simulink model "pid_C2000"  (R2018a)
settings: Solver=FixedStepDiscrete  StartTime=0.0  StopTime=Inf  RelTol=1e-3
undefined symbols (not defined in the file): Asymmetric, Up
libraries: c281xlib x2
settings Model: ExtModeTrigDuration=8  Creator=Administrator  LastModifiedBy=Administrator
settings SolverCC: AlgebraicLoopSolver=LineSearch
settings OptimizationCC: DefaultParameterBehavior=Inlined  UseDivisionForNetSlopeComputation=on  UseFloatMulNetSlope=on  DefaultUnderspecifiedDataType=single  InlineInvariantSignals=on  PassReuseOutputArgsAs=Individual arguments  ZeroExternalMemoryAtStartup=off  NoFixptDivByZeroProtection=on  EfficientFloat2IntCast=on  LifeSpan=1  MaxStackSize=512  OptimizeBlockOrder=speed  DifferentSizesBufferReuse=on
settings DebuggingCC: AlgebraicLoopMsg=none  ParameterTunabilityLossMsg=error
settings HardwareCC: ProdBitPerChar=16  ProdBitPerInt=16  ProdBitPerPointer=32  ProdBitPerSizeT=32  ProdBitPerPtrDiffT=32  ProdLargestAtomicInteger=Integer  ProdLargestAtomicFloat=None  ProdWordSize=16  ProdLongLongMode=on  ProdHWDeviceType=Texas Instruments->C2000
settings SFSimCC: MATLABDynamicMemAlloc=off
settings RTWCC: SystemTargetFile=ert.tlc  HardwareBoard=TI F281x  TLCOptions=-aInlineSetEventsForThisBaseRateFcn=TLC_FALSE -aSuppressMultiTaskScheduler=TLC_FALSE -aRateBasedStepFcn=1  TemplateMakefile=ert_default_tmf  GenerateReport=on  Toolchain=Texas Instruments Code Composer Studio (C2000)  IncludeHyperlinkInReport=on  LaunchReport=on  GenerateTraceInfo=on  GenerateTraceReport=on  GenerateTraceReportSl=on  GenerateTraceReportSf=on  GenerateTraceReportEml=on  GenerateCodeMetricsReport=on
settings CodeAppCC: ForceParamTrailComments=on  IgnoreCustomStorageClasses=off  OperatorAnnotations=on  SimulinkDataObjDesc=on  SFDataObjDesc=on  CustomSymbolStrGlobalVar=rt$N$M  CustomSymbolStrType=$N$M  CustomSymbolStrFcn=$N$M$F  CustomSymbolStrMacro=$N$M  InsertBlockDesc=on
settings ERTTargetCC: CodeReplacementLibrary=TI C28x  IncludeMdlTerminateFcn=off  CombineSignalStateStructs=on  SupportAbsoluteTime=off  SupportComplex=off  SupportNonInlinedSFcns=on  InlinedParameterPlacement=NonHierarchical  ERTFilePackagingFormat=CompactWithDataFile

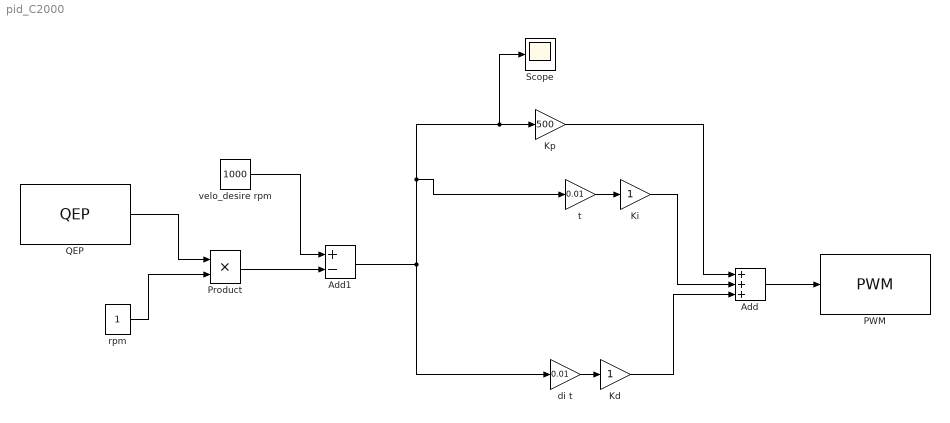
== system pid_C2000 ==
  Add : Sum  Inputs=+++
  Add1 : Sum  Inputs=+-
  Kd : Gain
  Ki : Gain
  Kp : Gain  Description=Kp  Gain=500
  PWM : c281xlib/PWM  useModule=A  timerSource=Specify via dialog  timerPeriod=37594  waveformType=Asymmetric(Up)  periodUnits=Clock cycles  preScaler=1/2  unit1Status=on  unit1Source=Input port  unit1Value=50  unit2Status=off  unit2Source=Specify via dialog  unit2Value=50  unit3Status=off  unit3Source=Specify via dialog  unit3Value=50  dutyCycleUnits=Clock cycles  logicSource=Specify via dialog  unit1_1Logic=Active low  unit1_2Logic=Active low  unit2_1Logic=Active high  unit2_2Logic=Active low  unit3_1Logic=Active high  unit3_2Logic=Active low  enableDeadband1=off  enableDeadband2=off  enableDeadband3=off  deadbandPrescaler=1  deadbandPeriodSource=Specify via dialog  deadbandPeriod=1  adcStartTrigger=None  adcstartEvent=None
      settings: SourceProductName=Embedded Coder Support Package for Texas Instruments C2000 Processors  SourceProductBaseCode=TIC2000
  Product : Product
  QEP : c281xlib/QEP  useModule=A  countingMode=RPM  positiveRotation=Clockwise  initialCount=0  encoderResolution=334  qepIndex=off  qepIndexQual=off  periodSource=Specify via dialog  period=65535  sampleTime=-1  dataType=uint16
      settings: SourceProductName=Embedded Coder Support Package for Texas Instruments C2000 Processors  SourceProductBaseCode=TIC2000
  Scope : Scope
  di t : Gain  Gain=0.01
  rpm : Constant
  t : Gain  Gain=0.01
  velo_desire rpm : Constant  Value=1000
  wires:
  velo_desire rpm/1 -> Add1/1
  Kp/1 -> Add/1
  Ki/1 -> Add/2
  Kd/1 -> Add/3
  t/1 -> Ki/1
  di t/1 -> Kd/1
  Add/1 -> PWM/1
  rpm/1 -> Product/2
  QEP/1 -> Product/1
  Product/1 -> Add1/2
  Add1/1 -> di t/1, t/1, Scope/1, Kp/1
